simulink model "lab11simulink"  (R2023b)
settings: Solver=VariableStepAuto  StartTime=0.0  StopTime=100  RelTol=1e-3
settings Model: Creator=mihai  LastModifiedBy=Cristi
settings DebuggingCC: UnconnectedInputMsg=warning  UnconnectedOutputMsg=warning  UnconnectedLineMsg=warning
settings ModelReferenceCC: EnableRefExpFcnMdlSchedulingChecks=on
settings RTWCC: DLArmComputeVersion=19.05

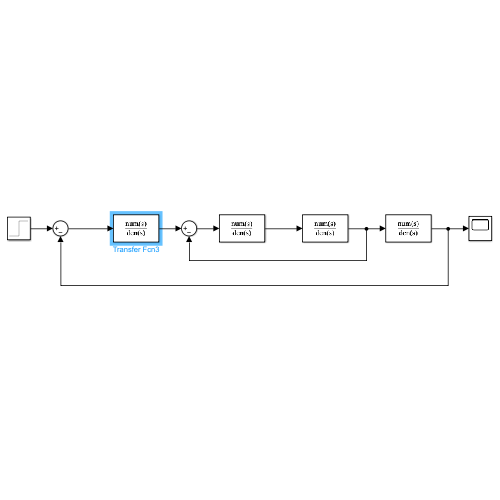
[thumbnail: Simulink's stored preview of the top-level diagram]
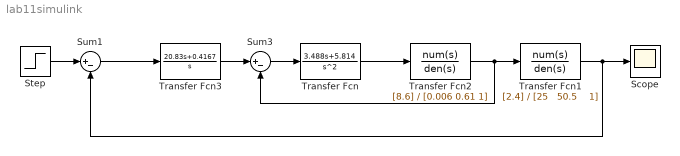
== system lab11simulink ==
  Scope : Scope
  Step : Step  SampleTime=0
  Sum1 : Sum  Inputs=|+-
  Sum3 : Sum  Inputs=|+-
  Transfer Fcn : TransferFcn  Numerator=[3.488 5.814]  Denominator=[1 0 0]
  Transfer Fcn1 : TransferFcn  Numerator=[2.4]  Denominator="[25   50.5    1]"
  Transfer Fcn2 : TransferFcn  Numerator=[8.6]  Denominator=[0.006 0.61 1]
  Transfer Fcn3 : TransferFcn  Numerator=[20.83 0.4167]  Denominator=[1 0]
  wires:
  Step/1 -> Sum1/1
  Transfer Fcn/1 -> Transfer Fcn2/1
  Sum1/1 -> Transfer Fcn3/1
  Sum3/1 -> Transfer Fcn/1
  Transfer Fcn3/1 -> Sum3/1
  Transfer Fcn2/1 -> Sum3/2, Transfer Fcn1/1
  Transfer Fcn1/1 -> Sum1/2, Scope/1
